simulink model "sys1"  (R2019a)
settings: Solver=ode4  StartTime=0.0  StopTime=100  FixedStep=0.01  RelTol=1e-3
InitFcn:
  | sys1Mec
values from neighbouring files (symbols this model uses):
  A = [-d/m  -k/m ... (first row only)    [sys1Mec.m]
  B = [1/m ; 0]    [sys1Mec.m]
  C = eye(2)    [sys1Mec.m]
  D = zeros(2,1)    [sys1Mec.m]
libraries: simulink x1
settings Model: Creator=alfyhack  LastModifiedBy=alfyhack

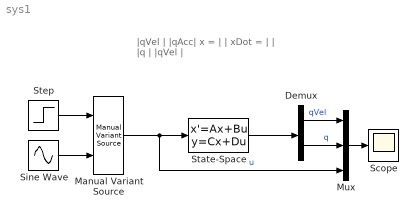
== system sys1 ==
  note: |qVel	|      		 	|qAcc|
      | x = |  	|	 xDot = 	|	  |
      |       |q	|        		|qVel |
  Demux : Demux  Outputs=2
  Manual Variant Source : simulink/Signal Routing/Manual Variant Source  NumChoices=2  LabelModeActiveChoice=V_1
      settings: SourceProductName=Simulink
  Mux : Mux  Inputs=3
  Scope : Scope
  Sine Wave : Sin  SampleTime=0
  State-Space : StateSpace  A=A  B=B  C=C  D=D  InitialCondition=0
  Step : Step  SampleTime=0
  wires:
  Step/1 -> Manual Variant Source/1
  Sine Wave/1 -> Manual Variant Source/2
  Manual Variant Source/1 -> Mux/3, State-Space/1  "u"
  State-Space/1 -> Demux/1
  Mux/1 -> Scope/1
  Demux/2 -> Mux/2  "q"
  Demux/1 -> Mux/1  "qVel"
